simulink library "general_sensor_lib"  (R2018b)
settings: Solver=ode45  StartTime=0.0  StopTime=10.0  RelTol=1e-3  EnableMultiTasking=on
libraries: simulink x3
settings Model: Creator=ge34qer  LastModifiedBy=ge34qer
settings DataIOCC: LimitDataPoints=on
settings OptimizationCC: LifeSpan=inf
settings DebuggingCC: AllowSymbolicDim=off  SFUnexpectedBacktrackingDiag=warning  SFNoUnconditionalDefaultTransitionDiag=warning
settings SFSimCC: SimUseLocalCustomCode=off
settings RTWCC: RTWUseLocalCustomCode=off
settings CodeAppCC: StateflowObjectComments=on
settings GRTTargetCC: TargetLangStandard=C89/C90 (ANSI)  GeneratePreprocessorConditionals=Disable all
settings ConfigComp: CovMetricSettings=dw  CovHtmlReporting=on  CovSaveCumulativeToWorkspaceVar=on  CovSaveSingleToWorkspaceVar=on  CovExternalEMLEnable=off

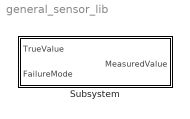
== system general_sensor_lib ==
  Subsystem : Subsystem  mask(Generic sensor model){Noise=0, Delay=0, SampleRate=0}
      mask help: A very generic sensor model which supports a specific sensor sample rate, a sensor delay and white noise.

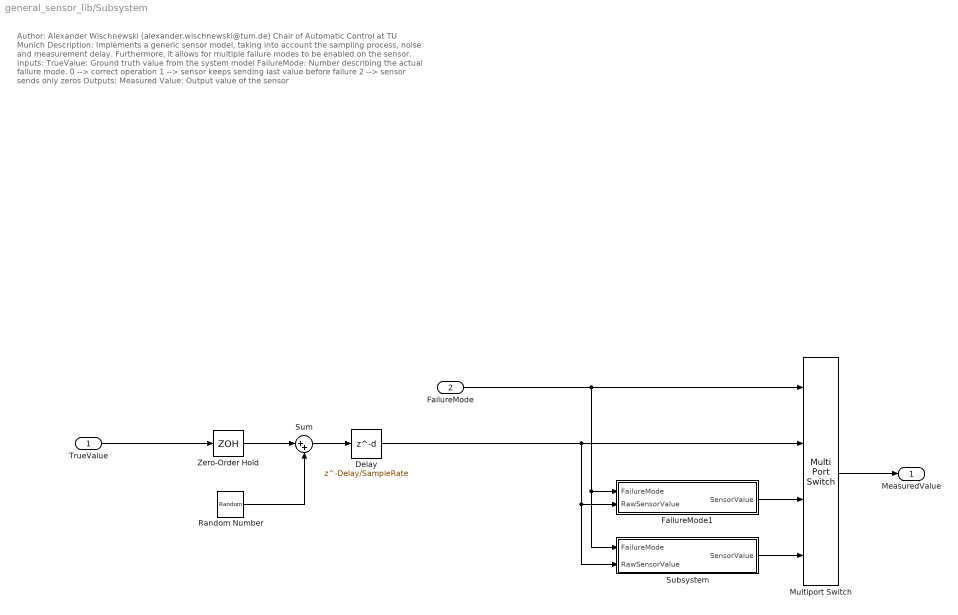
== system general_sensor_lib/Subsystem ==
  note: Author: Alexander Wischnewski (alexander.wischnewski@tum.de)
      | Chair of Automatic Control at TU Munich
      |
      | Description: Implements a generic sensor model, taking into account the sampling process, noise and measurement delay. Furthermore,
      | it allows for multiple failure modes to be enabled on the sensor.
      |
      | Inputs:
      | TrueValue: Ground truth value from the system model
      | FailureMode: Number describing the actual failure mode.
      | 0 --> correct operation
      | 1 --> sensor keeps sending last value before failure
      | 2 --> sensor sends only zeros
      |
      | Outputs:
      | Measured Value: Output value of the sensor
  TrueValue : Inport
  FailureMode : Inport  Port=2
  Delay : Delay  DelayLength=Delay/SampleRate  SampleTime=SampleRate
  FailureMode1 : Subsystem
  Multiport Switch : MultiPortSwitch  DataPortOrder=Zero-based contiguous  zeroidx=on
  Random Number : RandomNumber  Variance=Noise  SampleTime=SampleRate
  Subsystem : Subsystem
  Sum : Sum  Inputs=|++
  Zero-Order Hold : ZeroOrderHold  SampleTime=SampleRate
  MeasuredValue : Outport
  wires:
  Zero-Order Hold/1 -> Sum/1
  Random Number/1 -> Sum/2
  Sum/1 -> Delay/1
  TrueValue/1 -> Zero-Order Hold/1
  Delay/1 -> Multiport Switch/2, Subsystem/2(RawSensorValue), FailureMode1/2(RawSensorValue)
  Multiport Switch/1 -> MeasuredValue/1
  FailureMode/1 -> Subsystem/1(FailureMode), FailureMode1/1(FailureMode), Multiport Switch/1
  FailureMode1/1(SensorValue) -> Multiport Switch/3
  Subsystem/1(SensorValue) -> Multiport Switch/4

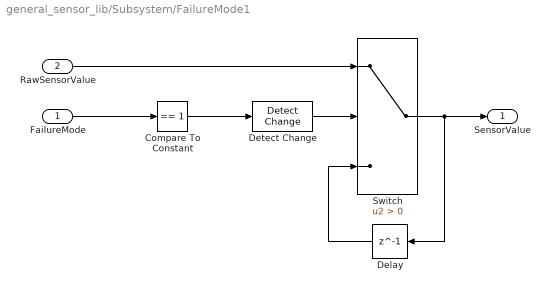
== system general_sensor_lib/Subsystem/FailureMode1 ==
  FailureMode : Inport
  RawSensorValue : Inport  Port=2
  Compare To Constant : simulink/Logic and Bit Operations/Compare To Constant  relop===  const=1  OutDataTypeStr=boolean
  Delay : Delay  DelayLength=1  InitialCondition=0
  Detect Change : simulink/Logic and Bit Operations/Detect Change  vinit=0  OutDataTypeStr=boolean
  Switch : Switch  Criteria=u2 > Threshold
  SensorValue : Outport
  wires:
  Switch/1 -> Delay/1, SensorValue/1
  Detect Change/1 -> Switch/2
  RawSensorValue/1 -> Switch/1
  Delay/1 -> Switch/3
  Compare To Constant/1 -> Detect Change/1
  FailureMode/1 -> Compare To Constant/1

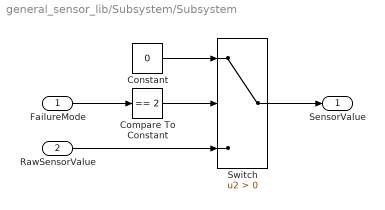
== system general_sensor_lib/Subsystem/Subsystem ==
  FailureMode : Inport
  RawSensorValue : Inport  Port=2
  Compare To Constant : simulink/Logic and Bit Operations/Compare To Constant  relop===  const=2  OutDataTypeStr=boolean
  Constant : Constant  Value=0
  Switch : Switch  Criteria=u2 > Threshold
  SensorValue : Outport
  wires:
  RawSensorValue/1 -> Switch/3
  FailureMode/1 -> Compare To Constant/1
  Compare To Constant/1 -> Switch/2
  Switch/1 -> SensorValue/1
  Constant/1 -> Switch/1
